simulink model "sampleModel2031"  (R2023a)
settings: Solver=VariableStepAuto  StartTime=0.0  StopTime=10.0  RelTol=1e-3
libraries: hdlsllib x9, simulink x2
settings Model: Creator=user1  LastModifiedBy=user1

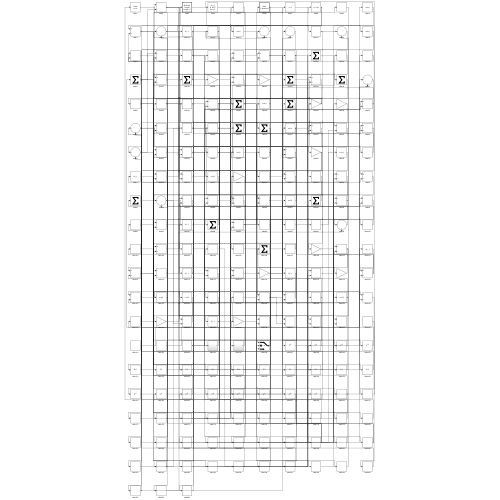
[thumbnail: Simulink's stored preview of the top-level diagram]
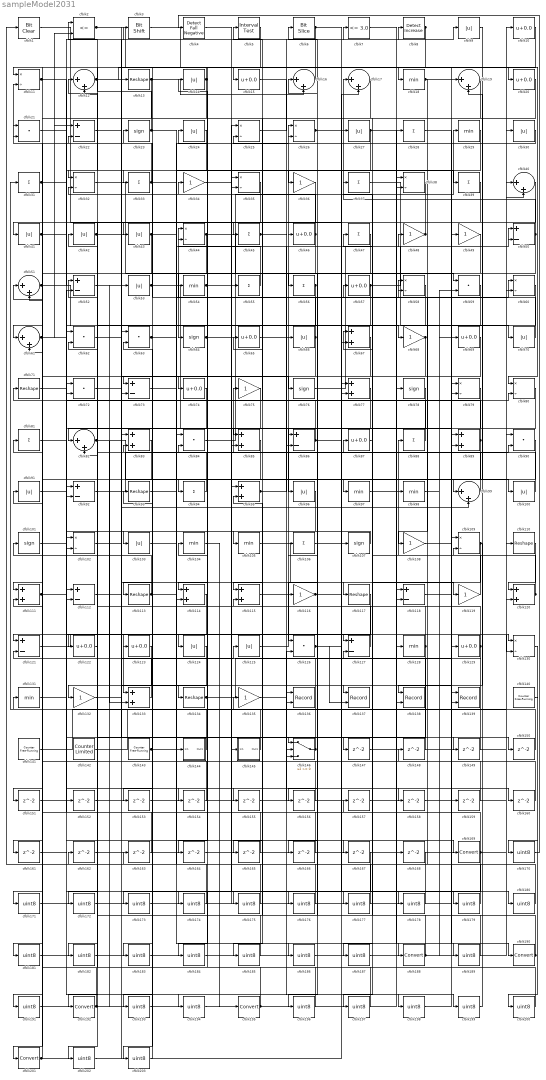
== system sampleModel2031 ==
  cfblk1 : simulink/Logic and Bit Operations/Bit Clear  iBit=0
      settings: LibrarySourceBlock=|
      | hdlsllib/Logic and Bit
      | Operations/Bit Clear
  cfblk{10,15,20,46,57,65,69,74,87,122..123,129} (12 alike) : Bias  Bias=0.0  SaturateOnIntegerOverflow=off
  cfblk{9,14,24,27,30,41..43,53,66,70,91,96,100,103,124..125} (17 alike) : Abs  SaturateOnIntegerOverflow=off
  cfblk{23,64,76,78,101,107} (6 alike) : Signum
  cfblk{11,25..26,32,35,38,44,58,60,79..80,102,109,130} (14 alike) : Product  Inputs=*/  RndMeth=Zero  SaturateOnIntegerOverflow=on
  cfblk{18,29,54,97..98,104..105,128,131} (9 alike) : MinMax
  cfblk{28,31,33,37,39,45,47,55..56,81,88,94,106} (13 alike) : Sum  Inputs=+
  cfblk{34,36,48..49,68,75,108,116,119,132,135} (11 alike) : Gain
  cfblk{13,71,93,110,113,117,134} (7 alike) : Reshape
  cfblk{67,77,83,85,89,95,111,114..115,120,133} (11 alike) : Sum
  cfblk{22,50,52,73,86,92,112,118,121,127} (10 alike) : Sum  Inputs=+-
  cfblk{12,16..17,19,40,51,61,82,99} (9 alike) : Sum  Inputs=|++
  cfblk{21,59,62..63,72,84,90,126} (8 alike) : DotProduct  OutDataTypeStr=Inherit: Inherit via internal rule
  cfblk136 : Record  FileSettingsInternal="{\"entries\":[{\"content\":{\"excelSettings\":{\"content\":{},\"type\":\"Streamout.ExcelSettings\"}},\"type\":\"Streamout.FileSettingStorage\",\"uuid\":\"\"}],\"packageUris\":[\"http:\\/\\/schema.mathworks.com\\/mf0\\/streamout_blocks\\/R2020a\"],\"version\":\"1.0\"}"  Layout=[1 1]  SignalsInternal="{\"entries\":[{\"content\":{\"signals\":[{\"content\":{\"blockPath\":[],\"dimensions\":[1],\"domain\":\"\",\"lineColor\":\"#a2142f\",\"plots\":[1],\"port\":1,\"signalID\":6125,\"signalName\":\"XY Graph:1\"},\"type\":\"RecordBlkView.Signal\",\"uuid\":\"\"},{\"content\":{\"blockPath\":[],\"dimensions\":[1],\"domain\":\"\",\"lineColor\":\"#139fff\",\"plots\":[1],\"port\":2,\"signalID\":6128,\"signalName\":\"XY Graph:2\"},\"type\":\"RecordBlkView.Signal\",\"uuid\":\"\"}]},\"type\":\"RecordBlkView.InputSignals\",\"uuid\":\"\"}],\"packageUris\":[\"http:\\/\\/schema.mathworks.com\\/mf0\\/streamout_blocks\\/R2020a\"],\"version\":\"1.0\"}"  VisualizationBindings="{\"xyplotplugin\":{\"info\":[{\"series\":[{\"bindingParametersList\":[{\"parameter\":\"X-Axis\",\"signalID\":6125,\"signalName\":\"XY Graph:1\"},{\"parameter\":\"Y-Axis\",\"signalID\":6128,\"signalName\":\"XY Graph:2\"}],\"seriesID\":37174}],\"subplotID\":1}]}}"  CompatibilityTag=XY  st=-1
  cfblk137 : Record  FileSettingsInternal="{\"entries\":[{\"content\":{\"excelSettings\":{\"content\":{},\"type\":\"Streamout.ExcelSettings\"}},\"type\":\"Streamout.FileSettingStorage\",\"uuid\":\"\"}],\"packageUris\":[\"http:\\/\\/schema.mathworks.com\\/mf0\\/streamout_blocks\\/R2020a\"],\"version\":\"1.0\"}"  Layout=[1 1]  SignalsInternal="{\"entries\":[{\"content\":{\"signals\":[{\"content\":{\"blockPath\":[],\"dimensions\":[1],\"domain\":\"\",\"lineColor\":\"#a2142f\",\"plots\":[1],\"port\":1,\"signalID\":6133,\"signalName\":\"XY Graph:1\"},\"type\":\"RecordBlkView.Signal\",\"uuid\":\"\"},{\"content\":{\"blockPath\":[],\"dimensions\":[1],\"domain\":\"\",\"lineColor\":\"#139fff\",\"plots\":[1],\"port\":2,\"signalID\":6136,\"signalName\":\"XY Graph:2\"},\"type\":\"RecordBlkView.Signal\",\"uuid\":\"\"}]},\"type\":\"RecordBlkView.InputSignals\",\"uuid\":\"\"}],\"packageUris\":[\"http:\\/\\/schema.mathworks.com\\/mf0\\/streamout_blocks\\/R2020a\"],\"version\":\"1.0\"}"  VisualizationBindings="{\"xyplotplugin\":{\"info\":[{\"series\":[{\"bindingParametersList\":[{\"parameter\":\"X-Axis\",\"signalID\":6133,\"signalName\":\"XY Graph:1\"},{\"parameter\":\"Y-Axis\",\"signalID\":6136,\"signalName\":\"XY Graph:2\"}],\"seriesID\":49207}],\"subplotID\":1}]}}"  CompatibilityTag=XY  st=-1
  cfblk138 : Record  FileSettingsInternal="{\"entries\":[{\"content\":{\"excelSettings\":{\"content\":{},\"type\":\"Streamout.ExcelSettings\"}},\"type\":\"Streamout.FileSettingStorage\",\"uuid\":\"\"}],\"packageUris\":[\"http:\\/\\/schema.mathworks.com\\/mf0\\/streamout_blocks\\/R2020a\"],\"version\":\"1.0\"}"  Layout=[1 1]  SignalsInternal="{\"entries\":[{\"content\":{\"signals\":[{\"content\":{\"blockPath\":[],\"dimensions\":[1],\"domain\":\"\",\"lineColor\":\"#a2142f\",\"plots\":[1],\"port\":1,\"signalID\":6141,\"signalName\":\"XY Graph:1\"},\"type\":\"RecordBlkView.Signal\",\"uuid\":\"\"},{\"content\":{\"blockPath\":[],\"dimensions\":[1],\"domain\":\"\",\"lineColor\":\"#139fff\",\"plots\":[1],\"port\":2,\"signalID\":6144,\"signalName\":\"XY Graph:2\"},\"type\":\"RecordBlkView.Signal\",\"uuid\":\"\"}]},\"type\":\"RecordBlkView.InputSignals\",\"uuid\":\"\"}],\"packageUris\":[\"http:\\/\\/schema.mathworks.com\\/mf0\\/streamout_blocks\\/R2020a\"],\"version\":\"1.0\"}"  VisualizationBindings="{\"xyplotplugin\":{\"info\":[{\"series\":[{\"bindingParametersList\":[{\"parameter\":\"X-Axis\",\"signalID\":6141,\"signalName\":\"XY Graph:1\"},{\"parameter\":\"Y-Axis\",\"signalID\":6144,\"signalName\":\"XY Graph:2\"}],\"seriesID\":27354}],\"subplotID\":1}]}}"  CompatibilityTag=XY  st=-1
  cfblk139 : Record  FileSettingsInternal="{\"entries\":[{\"content\":{\"excelSettings\":{\"content\":{},\"type\":\"Streamout.ExcelSettings\"}},\"type\":\"Streamout.FileSettingStorage\",\"uuid\":\"\"}],\"packageUris\":[\"http:\\/\\/schema.mathworks.com\\/mf0\\/streamout_blocks\\/R2020a\"],\"version\":\"1.0\"}"  Layout=[1 1]  SignalsInternal="{\"entries\":[{\"content\":{\"signals\":[{\"content\":{\"blockPath\":[],\"dimensions\":[1],\"domain\":\"\",\"lineColor\":\"#a2142f\",\"plots\":[1],\"port\":1,\"signalID\":6149,\"signalName\":\"XY Graph:1\"},\"type\":\"RecordBlkView.Signal\",\"uuid\":\"\"},{\"content\":{\"blockPath\":[],\"dimensions\":[1],\"domain\":\"\",\"lineColor\":\"#139fff\",\"plots\":[1],\"port\":2,\"signalID\":6152,\"signalName\":\"XY Graph:2\"},\"type\":\"RecordBlkView.Signal\",\"uuid\":\"\"}]},\"type\":\"RecordBlkView.InputSignals\",\"uuid\":\"\"}],\"packageUris\":[\"http:\\/\\/schema.mathworks.com\\/mf0\\/streamout_blocks\\/R2020a\"],\"version\":\"1.0\"}"  VisualizationBindings="{\"xyplotplugin\":{\"info\":[{\"series\":[{\"bindingParametersList\":[{\"parameter\":\"X-Axis\",\"signalID\":6149,\"signalName\":\"XY Graph:1\"},{\"parameter\":\"Y-Axis\",\"signalID\":6152,\"signalName\":\"XY Graph:2\"}],\"seriesID\":25762}],\"subplotID\":1}]}}"  CompatibilityTag=XY  st=-1
  cfblk140 : hdlsllib/Sources/Counter Free-Running  NumBits=16  tsamp=-1
  cfblk141 : hdlsllib/Sources/Counter Free-Running  NumBits=16  tsamp=-1
  cfblk142 : hdlsllib/Sources/Counter Limited  uplimit=7  tsamp=-1
  cfblk143 : hdlsllib/Sources/Counter Free-Running  NumBits=16  tsamp=-1
  cfblk144 : Subsystem
      settings: LibrarySourceBlock=|
      | hdlsllib/Ports &
      | Subsystems/Subsystem
  cfblk145 : Subsystem
      settings: LibrarySourceBlock=|
      | hdlsllib/Ports &
      | Subsystems/Subsystem
  cfblk146 : Switch  SaturateOnIntegerOverflow=off  InputSameDT=off
  cfblk{147..168} (22 alike) : Delay  SampleTime=1
  cfblk{169,188,190,192,195,201} (6 alike) : DataTypeConversion  SaturateOnIntegerOverflow=off  RndMeth=Floor
  cfblk{170..187,189,191,193..194,196..200,202..203} (29 alike) : DataTypeConversion  OutDataTypeStr=uint8  SaturateOnIntegerOverflow=off  RndMeth=Floor
  cfblk2 : RelationalOperator  Operator=<=  OutDataTypeStr=boolean  InputSameDT=off
  cfblk3 : hdlsllib/Logic and Bit Operations/Bit Shift  mode=Shift Left Logical  N=0
  cfblk4 : hdlsllib/Logic and Bit Operations/Detect Fall Negative  vinit=0  OutDataTypeStr=boolean
  cfblk5 : hdlsllib/Logic and Bit Operations/Interval Test  IntervalClosedRight=on  uplimit=0.5  IntervalClosedLeft=on  lowlimit=-0.5  OutDataTypeStr=boolean
  cfblk6 : hdlsllib/Logic and Bit Operations/Bit Slice  lidx=7  ridx=0
  cfblk7 : hdlsllib/Logic and Bit Operations/Compare To Constant  relop=<=  const=3.0  OutDataTypeStr=boolean
  cfblk8 : simulink/Logic and Bit Operations/Detect Increase  vinit=0.0  OutDataTypeStr=boolean
      settings: LibrarySourceBlock=|
      | hdlsllib/Logic and Bit
      | Operations/Detect
      | Increase
  wires:
  cfblk38/1 -> cfblk192/1
  cfblk125/1 -> cfblk26/1
  cfblk77/1 -> cfblk96/1
  cfblk87/1 -> cfblk47/1
  cfblk70/1 -> cfblk23/1
  cfblk37/1 -> cfblk70/1
  cfblk84/1 -> cfblk29/1
  cfblk76/1 -> cfblk48/1
  cfblk57/1 -> cfblk30/1, cfblk86/2
  cfblk102/1 -> cfblk13/1
  cfblk12/1 -> cfblk80/1, cfblk114/2
  cfblk98/1 -> cfblk69/1
  cfblk128/1 -> cfblk37/1, cfblk202/1
  cfblk31/1 -> cfblk22/1, cfblk67/2, cfblk175/1
  cfblk105/1 -> cfblk117/1
  cfblk14/1 -> cfblk11/1, cfblk43/1
  cfblk119/1 -> cfblk88/1
  cfblk127/1 -> cfblk16/1
  cfblk4/1 -> cfblk169/1
  cfblk66/1 -> cfblk94/1, cfblk44/2
  cfblk86/1 -> cfblk5/1, cfblk160/1
  cfblk111/1 -> cfblk154/1, cfblk199/1
  cfblk36/1 -> cfblk134/1
  cfblk109/1 -> cfblk138/1, cfblk187/1
  cfblk135/1 -> cfblk188/1
  cfblk64/1 -> cfblk57/1, cfblk179/1
  cfblk28/1 -> cfblk190/1
  cfblk3/1 -> cfblk18/1
  cfblk117/1 -> cfblk133/1
  cfblk25/1 -> cfblk9/1
  cfblk53/1 -> cfblk98/1, cfblk46/1
  cfblk122/1 -> cfblk31/1
  cfblk69/1 -> cfblk82/1
  cfblk60/1 -> cfblk73/1
  cfblk94/1 -> cfblk71/1
  cfblk43/1 -> cfblk85/2, cfblk161/1
  cfblk52/1 -> cfblk68/1
  cfblk100/1 -> cfblk75/1
  cfblk123/1 -> cfblk132/1
  cfblk63/1 -> cfblk144/1(In1), cfblk130/2
  cfblk2/1 -> cfblk55/1, cfblk76/1, cfblk138/2
  cfblk74/1 -> cfblk82/2
  cfblk56/1 -> cfblk114/1, cfblk73/2
  cfblk81/1 -> cfblk80/2
  cfblk62/1 -> cfblk7/1
  cfblk82/1 -> cfblk97/1, cfblk133/2
  cfblk44/1 -> cfblk139/1, cfblk100/1, cfblk153/1
  cfblk9/1 -> cfblk99/1
  cfblk8/1 -> cfblk111/1, cfblk164/1
  cfblk61/1 -> cfblk92/2, cfblk2/2
  cfblk110/1 -> cfblk120/1
  cfblk47/1 -> cfblk105/1
  cfblk58/1 -> cfblk146/1
  cfblk6/1 -> cfblk130/1, cfblk33/1
  cfblk23/1 -> cfblk56/1, cfblk2/1, cfblk39/1
  cfblk29/1 -> cfblk85/1
  cfblk145/1(Out1) -> cfblk81/1
  cfblk1/1 -> cfblk77/2
  cfblk42/1 -> cfblk64/1, cfblk137/1
  cfblk20/1 -> cfblk121/1
  cfblk113/1 -> cfblk90/2, cfblk21/1
  cfblk133/1 -> cfblk12/1
  cfblk92/1 -> cfblk40/2
  cfblk33/1 -> cfblk11/2, cfblk36/1
  cfblk83/1 -> cfblk201/1
  cfblk13/1 -> cfblk16/2, cfblk61/1
  cfblk46/1 -> cfblk74/1, cfblk22/2
  cfblk16/1 -> cfblk15/1
  cfblk73/1 -> cfblk26/2
  cfblk15/1 -> cfblk136/1
  cfblk142/1 -> cfblk10/1
  cfblk32/1 -> cfblk145/1(In1)
  cfblk132/1 -> cfblk125/1
  cfblk45/1 -> cfblk139/2, cfblk177/1
  cfblk146/1 -> cfblk95/2, cfblk93/1
  cfblk91/1 -> cfblk127/1
  cfblk120/1 -> cfblk109/2, cfblk67/1
  cfblk24/1 -> cfblk72/2
  cfblk121/1 -> cfblk123/1
  cfblk116/1 -> cfblk58/1, cfblk17/2
  cfblk40/1 -> cfblk115/1
  cfblk41/1 -> cfblk112/1, cfblk146/3
  cfblk103/1 -> cfblk119/1
  cfblk115/1 -> cfblk126/1
  cfblk108/1 -> cfblk129/1
  cfblk104/1 -> cfblk195/1
  cfblk59/1 -> cfblk122/1
  cfblk50/1 -> cfblk17/1, cfblk166/1
  cfblk72/1 -> cfblk8/1
  cfblk27/1 -> cfblk113/1, cfblk89/2
  cfblk11/1 -> cfblk86/1, cfblk158/1
  cfblk39/1 -> cfblk112/2
  cfblk143/1 -> cfblk60/1, cfblk50/1
  cfblk141/1 -> cfblk60/2
  cfblk54/1 -> cfblk25/1, cfblk136/2
  cfblk96/1 -> cfblk102/2
  cfblk51/1 -> cfblk78/1, cfblk3/1
  cfblk48/1 -> cfblk45/1, cfblk41/1
  cfblk134/1 -> cfblk89/1, cfblk54/1
  cfblk99/1 -> cfblk12/2
  cfblk88/1 -> cfblk51/1
  cfblk89/1 -> cfblk65/1, cfblk124/1
  cfblk18/1 -> cfblk20/1, cfblk108/1
  cfblk107/1 -> cfblk103/1
  cfblk126/1 -> cfblk27/1, cfblk137/2
  cfblk129/1 -> cfblk52/1, cfblk127/2
  cfblk55/1 -> cfblk44/1
  cfblk112/1 -> cfblk99/2
  cfblk7/1 -> cfblk128/1
  cfblk68/1 -> cfblk116/1, cfblk151/1
  cfblk10/1 -> cfblk32/1
  cfblk144/1(Out1) -> cfblk101/1
  cfblk26/1 -> cfblk59/1, cfblk150/1
  cfblk95/1 -> cfblk66/1, cfblk50/2
  cfblk30/1 -> cfblk25/2
  cfblk78/1 -> cfblk147/1
  cfblk147/1 -> cfblk90/1
  cfblk148/1 -> cfblk62/1
  cfblk22/1 -> cfblk149/1
  cfblk149/1 -> cfblk121/2
  cfblk150/1 -> cfblk115/2
  cfblk151/1 -> cfblk52/2
  cfblk71/1 -> cfblk152/1
  cfblk152/1 -> cfblk40/1
  cfblk153/1 -> cfblk126/2
  cfblk154/1 -> cfblk102/1
  cfblk101/1 -> cfblk155/1
  cfblk155/1 -> cfblk146/2
  cfblk80/1 -> cfblk156/1
  cfblk156/1 -> cfblk95/1
  cfblk157/1 -> cfblk109/1
  cfblk158/1 -> cfblk58/2
  cfblk159/1 -> cfblk111/2
  cfblk160/1 -> cfblk61/2
  cfblk162/1 -> cfblk77/1
  cfblk163/1 -> cfblk72/1
  cfblk164/1 -> cfblk120/2
  cfblk17/1 -> cfblk165/1
  cfblk165/1 -> cfblk92/1
  cfblk166/1 -> cfblk51/2
  cfblk21/1 -> cfblk167/1
  cfblk168/1 -> cfblk1/1
  cfblk169/1 -> cfblk42/1, cfblk184/1
  cfblk130/1 -> cfblk170/1
  cfblk170/1 -> cfblk4/1
  cfblk35/1 -> cfblk171/1
  cfblk171/1 -> cfblk159/1
  cfblk124/1 -> cfblk172/1
  cfblk172/1 -> cfblk35/1
  cfblk5/1 -> cfblk173/1
  cfblk173/1 -> cfblk35/2
  cfblk131/1 -> cfblk174/1
  cfblk174/1 -> cfblk84/1
  cfblk175/1 -> cfblk131/1
  cfblk34/1 -> cfblk176/1
  cfblk176/1 -> cfblk84/2
  cfblk177/1 -> cfblk34/1
  cfblk106/1 -> cfblk178/1
  cfblk178/1 -> cfblk162/1
  cfblk179/1 -> cfblk106/1
  cfblk118/1 -> cfblk180/1
  cfblk180/1 -> cfblk148/1
  cfblk67/1 -> cfblk181/1
  cfblk181/1 -> cfblk118/1
  cfblk85/1 -> cfblk182/1
  cfblk182/1 -> cfblk118/2
  cfblk49/1 -> cfblk183/1
  cfblk183/1 -> cfblk163/1
  cfblk184/1 -> cfblk49/1
  cfblk79/1 -> cfblk185/1
  cfblk185/1 -> cfblk24/1
  cfblk93/1 -> cfblk186/1
  cfblk186/1 -> cfblk79/1
  cfblk187/1 -> cfblk79/2
  cfblk188/1 -> cfblk32/2, cfblk87/1, cfblk59/2, cfblk6/1, cfblk110/1
  cfblk97/1 -> cfblk189/1
  cfblk189/1 -> cfblk135/1
  cfblk190/1 -> cfblk157/1, cfblk14/1
  cfblk114/1 -> cfblk191/1
  cfblk191/1 -> cfblk28/1
  cfblk192/1 -> cfblk91/1, cfblk53/1
  cfblk75/1 -> cfblk193/1
  cfblk193/1 -> cfblk38/1
  cfblk161/1 -> cfblk194/1
  cfblk194/1 -> cfblk38/2
  cfblk195/1 -> cfblk168/1, cfblk62/2
  cfblk90/1 -> cfblk196/1
  cfblk196/1 -> cfblk104/1
  cfblk19/1 -> cfblk197/1
  cfblk197/1 -> cfblk63/1
  cfblk65/1 -> cfblk198/1
  cfblk198/1 -> cfblk19/1
  cfblk199/1 -> cfblk19/2
  cfblk140/1 -> cfblk200/1
  cfblk200/1 -> cfblk63/2
  cfblk201/1 -> cfblk21/2, cfblk107/1
  cfblk202/1 -> cfblk83/1
  cfblk167/1 -> cfblk203/1
  cfblk203/1 -> cfblk83/2

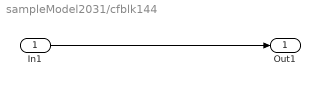
== system sampleModel2031/cfblk144 ==
  In1 : Inport
  Out1 : Outport
  wires:
  In1/1 -> Out1/1

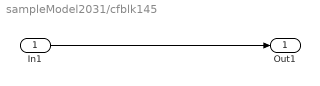
== system sampleModel2031/cfblk145 ==
  In1 : Inport
  Out1 : Outport
  wires:
  In1/1 -> Out1/1
